simulink model "sampleModel1859"  (R2023a)
settings: Solver=VariableStepAuto  StartTime=0.0  StopTime=10.0  RelTol=1e-3
libraries: hdlsllib x5, simulink x2
settings Model: Creator=user1  LastModifiedBy=user1

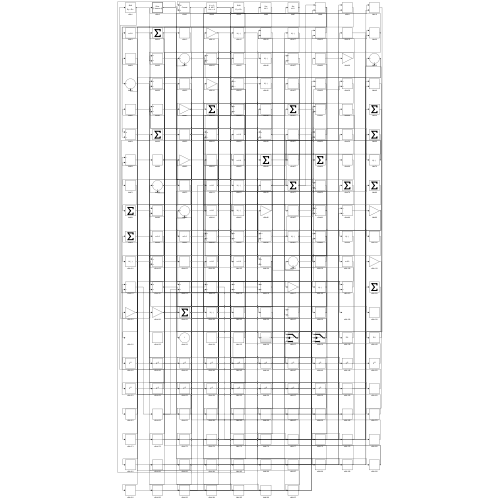
[thumbnail: Simulink's stored preview of the top-level diagram]
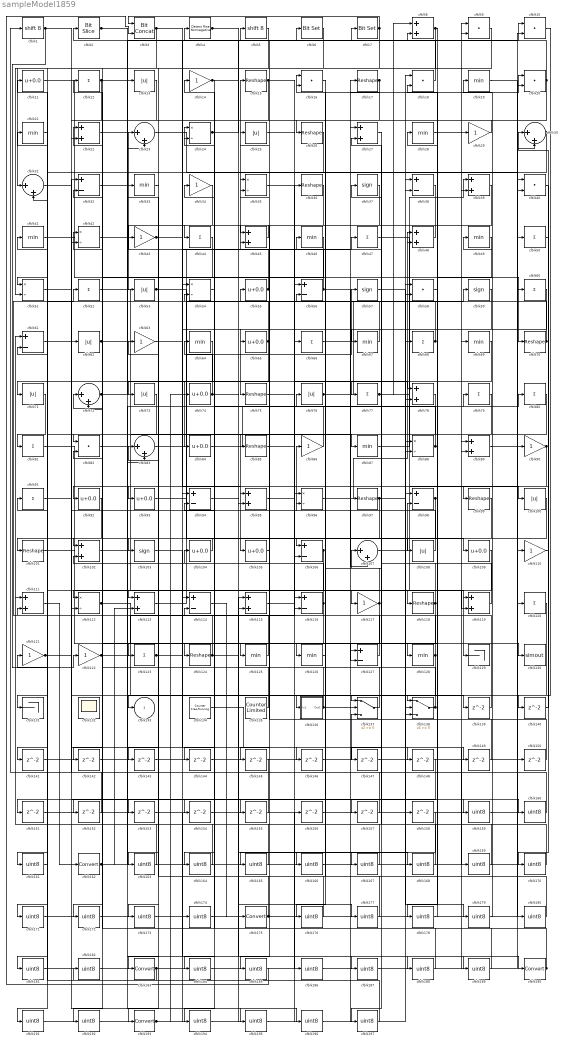
== system sampleModel1859 ==
  cfblk1 : ArithShift  BitShiftNumber=8
  cfblk{9..10,16,18,20,40,58,82} (8 alike) : DotProduct  OutDataTypeStr=Inherit: Inherit via internal rule
  cfblk{13,25,53,62,71,73,76,100,108} (9 alike) : Abs  SaturateOnIntegerOverflow=off
  cfblk{15,17,26,36,70,75,85,97,99,101,118,124} (12 alike) : Reshape
  cfblk{8,22,27,39,45,48,78,89,95,102,111,113,115,119} (14 alike) : Sum
  cfblk{37,57,59,103} (4 alike) : Signum
  cfblk{11,55,65,74,84,92..93,104..105,109} (10 alike) : Bias  Bias=0.0  SaturateOnIntegerOverflow=off
  cfblk{32,38,56,61,94,98,106,114,116,127} (10 alike) : Sum  Inputs=+-
  cfblk{23,30..31,72,83,107} (6 alike) : Sum  Inputs=|++
  cfblk{14,29,34,43,63,86,90,110,117,121..122} (11 alike) : Gain
  cfblk{24,35,42,51,54,88,96,112} (8 alike) : Product  Inputs=*/  RndMeth=Zero  SaturateOnIntegerOverflow=on
  cfblk{12,44,47,50,52,60,66,68,77,79..81,91,120,123} (15 alike) : Sum  Inputs=+
  cfblk{19,21,28,33,41,46,49,64,67,69,87,125..126,128} (14 alike) : MinMax
  cfblk129 : Terminator
  cfblk130 : ToWorkspace  VariableName=simout  SaveFormat=Timeseries  SampleTime=-1
  cfblk131 : Terminator
  cfblk132 : Scope
      settings: Floating=on
  cfblk134 : hdlsllib/Sources/Counter Free-Running  NumBits=16  tsamp=-1
  cfblk135 : hdlsllib/Sources/Counter Limited  uplimit=7  tsamp=-1
  cfblk136 : Subsystem
      settings: LibrarySourceBlock=|
      | hdlsllib/Ports &
      | Subsystems/Subsystem
  cfblk137 : Switch  SaturateOnIntegerOverflow=off  InputSameDT=off
  cfblk138 : Switch  SaturateOnIntegerOverflow=off  InputSameDT=off
  cfblk{139..158} (20 alike) : Delay  SampleTime=1
  cfblk{159..161,163..174,176..182,184..189,191..192,194..197} (34 alike) : DataTypeConversion  OutDataTypeStr=uint8  SaturateOnIntegerOverflow=off  RndMeth=Floor
  cfblk{162,175,183,190,193} (5 alike) : DataTypeConversion  SaturateOnIntegerOverflow=off  RndMeth=Floor
  cfblk2 : hdlsllib/Logic and Bit Operations/Bit Slice  lidx=7  ridx=0
  cfblk3 : hdlsllib/Logic and Bit Operations/Bit Concat  numInputs=2
  cfblk4 : hdlsllib/Logic and Bit Operations/Detect Rise Nonnegative  vinit=0  OutDataTypeStr=boolean
  cfblk5 : ArithShift  BitShiftNumber=8
  cfblk6 : simulink/Logic and Bit Operations/Bit Set  iBit=0
      settings: LibrarySourceBlock=|
      | hdlsllib/Logic and Bit
      | Operations/Bit Set
  cfblk7 : simulink/Logic and Bit Operations/Bit Set  iBit=0
      settings: LibrarySourceBlock=|
      | hdlsllib/Logic and Bit
      | Operations/Bit Set
  cfblk133 : Outport  VectorParamsAs1DForOutWhenUnconnected=off
  wires:
  cfblk45/1 -> cfblk44/1
  cfblk119/1 -> cfblk46/1
  cfblk101/1 -> cfblk117/1
  cfblk37/1 -> cfblk71/1
  cfblk127/1 -> cfblk52/1
  cfblk83/1 -> cfblk59/1
  cfblk20/1 -> cfblk2/1, cfblk73/1
  cfblk40/1 -> cfblk99/1
  cfblk78/1 -> cfblk105/1
  cfblk113/1 -> cfblk36/1
  cfblk56/1 -> cfblk23/1, cfblk107/2
  cfblk52/1 -> cfblk118/1
  cfblk16/1 -> cfblk126/1
  cfblk7/1 -> cfblk3/1, cfblk93/1
  cfblk24/1 -> cfblk6/1, cfblk168/1
  cfblk100/1 -> cfblk103/1
  cfblk11/1 -> cfblk70/1
  cfblk87/1 -> cfblk39/1
  cfblk71/1 -> cfblk81/1
  cfblk67/1 -> cfblk22/1
  cfblk53/1 -> cfblk106/1, cfblk65/1
  cfblk26/1 -> cfblk82/1
  cfblk10/1 -> cfblk137/1
  cfblk117/1 -> cfblk16/1, cfblk143/1
  cfblk14/1 -> cfblk124/1, cfblk116/2
  cfblk35/1 -> cfblk109/1
  cfblk33/1 -> cfblk113/1
  cfblk98/1 -> cfblk138/2, cfblk197/1
  cfblk17/1 -> cfblk16/2, cfblk164/1
  cfblk62/1 -> cfblk87/1, cfblk188/1
  cfblk138/1 -> cfblk63/1, cfblk82/2
  cfblk15/1 -> cfblk66/1, cfblk72/2
  cfblk135/1 -> cfblk83/1
  cfblk96/1 -> cfblk48/1
  cfblk55/1 -> cfblk15/1, cfblk43/1
  cfblk74/1 -> cfblk64/1, cfblk177/1
  cfblk28/1 -> cfblk29/1
  cfblk77/1 -> cfblk129/1, cfblk8/1
  cfblk68/1 -> cfblk55/1, cfblk67/1
  cfblk43/1 -> cfblk95/1, cfblk153/1
  cfblk105/1 -> cfblk35/1
  cfblk108/1 -> cfblk86/1
  cfblk120/1 -> cfblk183/1
  cfblk18/1 -> cfblk4/1
  cfblk25/1 -> cfblk96/1
  cfblk4/1 -> cfblk146/1, cfblk160/1
  cfblk95/1 -> cfblk47/1
  cfblk41/1 -> cfblk116/1
  cfblk29/1 -> cfblk26/1
  cfblk70/1 -> cfblk19/1, cfblk5/1
  cfblk51/1 -> cfblk62/1
  cfblk5/1 -> cfblk31/1
  cfblk58/1 -> cfblk28/1
  cfblk34/1 -> cfblk53/1
  cfblk93/1 -> cfblk57/1
  cfblk47/1 -> cfblk100/1
  cfblk66/1 -> cfblk48/2
  cfblk121/1 -> cfblk21/1, cfblk96/2
  cfblk48/1 -> cfblk45/1
  cfblk84/1 -> cfblk79/1
  cfblk128/1 -> cfblk42/1, cfblk25/1, cfblk147/1
  cfblk8/1 -> cfblk128/1, cfblk95/2, cfblk31/2
  cfblk81/1 -> cfblk130/1
  cfblk1/1 -> cfblk122/1, cfblk138/3
  cfblk23/1 -> cfblk90/1
  cfblk54/1 -> cfblk24/1
  cfblk111/1 -> cfblk162/1
  cfblk123/1 -> cfblk45/2, cfblk10/1
  cfblk59/1 -> cfblk75/1
  cfblk21/1 -> cfblk51/1
  cfblk76/1 -> cfblk39/2, cfblk20/1
  cfblk12/1 -> cfblk22/2, cfblk136/1(In1)
  cfblk106/1 -> cfblk123/1, cfblk191/1
  cfblk104/1 -> cfblk101/1
  cfblk13/1 -> cfblk92/1
  cfblk97/1 -> cfblk68/1, cfblk154/1
  cfblk64/1 -> cfblk84/1
  cfblk69/1 -> cfblk106/2
  cfblk90/1 -> cfblk102/1, cfblk133/1
  cfblk137/1 -> cfblk104/1
  cfblk124/1 -> cfblk12/1, cfblk157/1
  cfblk65/1 -> cfblk41/1, cfblk112/2
  cfblk115/1 -> cfblk190/1
  cfblk75/1 -> cfblk119/1
  cfblk125/1 -> cfblk11/1
  cfblk136/1(Out1) -> cfblk32/2, cfblk139/1
  cfblk88/1 -> cfblk54/2, cfblk108/1
  cfblk107/1 -> cfblk98/2
  cfblk30/1 -> cfblk42/2, cfblk141/1
  cfblk72/1 -> cfblk112/1, cfblk8/2
  cfblk86/1 -> cfblk24/2
  cfblk118/1 -> cfblk37/1, cfblk184/1
  cfblk63/1 -> cfblk7/1
  cfblk102/1 -> cfblk80/1
  cfblk3/1 -> cfblk85/1, cfblk51/2
  cfblk114/1 -> cfblk175/1
  cfblk116/1 -> cfblk72/1, cfblk192/1
  cfblk38/1 -> cfblk193/1
  cfblk112/1 -> cfblk127/2, cfblk152/1
  cfblk82/1 -> cfblk119/2
  cfblk80/1 -> cfblk131/1
  cfblk22/1 -> cfblk23/2
  cfblk42/1 -> cfblk13/1
  cfblk2/1 -> cfblk77/1, cfblk125/1
  cfblk122/1 -> cfblk56/1, cfblk138/1
  cfblk32/1 -> cfblk78/1
  cfblk139/1 -> cfblk107/1
  cfblk110/1 -> cfblk140/1
  cfblk140/1 -> cfblk30/1
  cfblk141/1 -> cfblk78/2
  cfblk46/1 -> cfblk142/1
  cfblk39/1 -> cfblk144/1
  cfblk144/1 -> cfblk137/2
  cfblk36/1 -> cfblk145/1
  cfblk145/1 -> cfblk1/1
  cfblk146/1 -> cfblk137/3
  cfblk147/1 -> cfblk10/2
  cfblk103/1 -> cfblk148/1
  cfblk31/1 -> cfblk149/1
  cfblk149/1 -> cfblk127/1
  cfblk19/1 -> cfblk150/1
  cfblk150/1 -> cfblk35/2
  cfblk73/1 -> cfblk151/1
  cfblk151/1 -> cfblk98/1
  cfblk152/1 -> cfblk32/1
  cfblk154/1 -> cfblk40/2
  cfblk79/1 -> cfblk155/1
  cfblk155/1 -> cfblk54/1
  cfblk156/1 -> cfblk88/2
  cfblk157/1 -> cfblk56/2
  cfblk61/1 -> cfblk159/1
  cfblk159/1 -> cfblk110/1
  cfblk160/1 -> cfblk61/1
  cfblk92/1 -> cfblk161/1
  cfblk161/1 -> cfblk61/2
  cfblk162/1 -> cfblk83/2, cfblk113/2, cfblk69/1
  cfblk143/1 -> cfblk163/1
  cfblk163/1 -> cfblk111/1
  cfblk164/1 -> cfblk111/2
  cfblk60/1 -> cfblk165/1
  cfblk165/1 -> cfblk121/1
  cfblk126/1 -> cfblk166/1
  cfblk166/1 -> cfblk60/1
  cfblk27/1 -> cfblk167/1
  cfblk167/1 -> cfblk14/1
  cfblk168/1 -> cfblk27/1
  cfblk134/1 -> cfblk169/1
  cfblk169/1 -> cfblk27/2
  cfblk50/1 -> cfblk170/1
  cfblk170/1 -> cfblk34/1
  cfblk6/1 -> cfblk171/1
  cfblk171/1 -> cfblk50/1
  cfblk9/1 -> cfblk172/1
  cfblk172/1 -> cfblk30/2
  cfblk44/1 -> cfblk173/1
  cfblk173/1 -> cfblk9/1
  cfblk174/1 -> cfblk9/2
  cfblk175/1 -> cfblk20/2, cfblk58/2, cfblk97/1, cfblk33/1
  cfblk99/1 -> cfblk176/1
  cfblk176/1 -> cfblk114/1
  cfblk177/1 -> cfblk114/2
  cfblk49/1 -> cfblk178/1
  cfblk178/1 -> cfblk18/2
  cfblk57/1 -> cfblk179/1
  cfblk179/1 -> cfblk49/1
  cfblk89/1 -> cfblk180/1
  cfblk180/1 -> cfblk76/1
  cfblk148/1 -> cfblk181/1
  cfblk181/1 -> cfblk89/1
  cfblk182/1 -> cfblk89/2
  cfblk183/1 -> cfblk182/1, cfblk18/1
  cfblk184/1 -> cfblk120/1
  cfblk158/1 -> cfblk185/1
  cfblk185/1 -> cfblk3/2
  cfblk85/1 -> cfblk186/1
  cfblk186/1 -> cfblk158/1
  cfblk94/1 -> cfblk187/1
  cfblk187/1 -> cfblk40/1
  cfblk188/1 -> cfblk94/1
  cfblk153/1 -> cfblk189/1
  cfblk189/1 -> cfblk94/2
  cfblk190/1 -> cfblk102/2, cfblk58/1
  cfblk191/1 -> cfblk115/1
  cfblk192/1 -> cfblk115/2
  cfblk193/1 -> cfblk174/1, cfblk156/1, cfblk74/1, cfblk17/1
  cfblk109/1 -> cfblk194/1
  cfblk194/1 -> cfblk38/1
  cfblk142/1 -> cfblk195/1
  cfblk195/1 -> cfblk38/2
  cfblk91/1 -> cfblk196/1
  cfblk196/1 -> cfblk88/1
  cfblk197/1 -> cfblk91/1

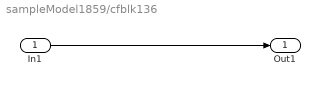
== system sampleModel1859/cfblk136 ==
  In1 : Inport
  Out1 : Outport
  wires:
  In1/1 -> Out1/1
